simulink model "prova"  (R2018b)
settings: Solver=VariableStepAuto  StartTime=0.0  StopTime=inf  RelTol=1e-3
libraries: robotlib x3
settings Model: Creator=francesco  LastModifiedBy=francesco

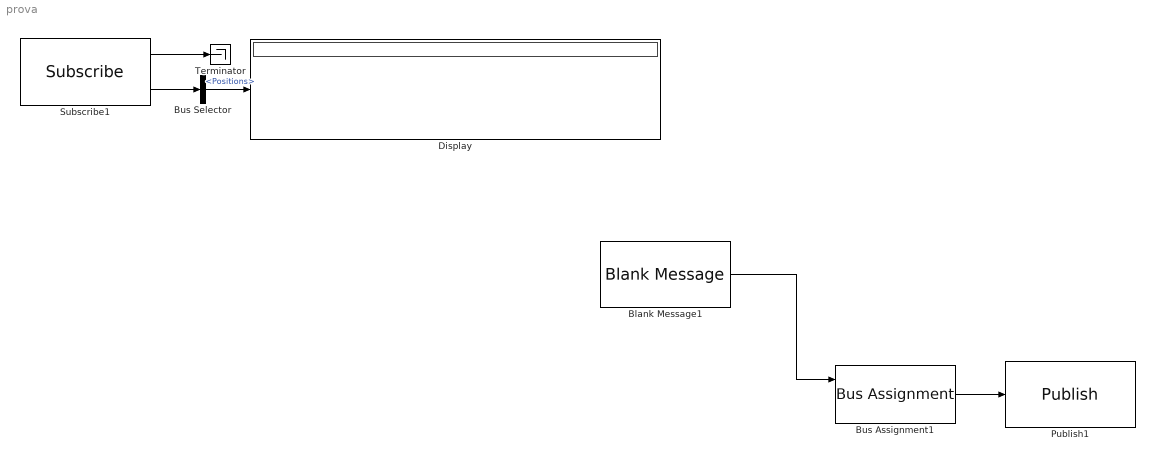
== system prova ==
  Blank Message1 : robotlib/Blank Message  messageClass=Message  entityType=std_msgs/Float64  messageType=std_msgs/Float64  SampleTime=-1
      settings: SourceProductBaseCode=RO
  Bus Assignment1 : BusAssignment  AssignedSignals=Data
  Bus Selector : BusSelector  OutputSignals=Actual.Positions
  Display : Display
  Publish1 : robotlib/Publish  topicSource=Select from ROS network  topic=/arm_controller/state  messageType=control_msgs/JointTrajectoryControllerState  messageQueueLength=1
      settings: SourceProductBaseCode=RO
  Subscribe1 : robotlib/Subscribe  topicSource=Select from ROS network  topic=/arm_controller/state  messageType=control_msgs/JointTrajectoryControllerState  sampleTime=-1  messageQueueLength=1
      settings: SourceProductBaseCode=RO
  Terminator : Terminator
  wires:
  Subscribe1/2 -> Bus Selector/1
  Subscribe1/1 -> Terminator/1
  Bus Assignment1/1 -> Publish1/1
  Blank Message1/1 -> Bus Assignment1/1
  Bus Selector/1 -> Display/1  "<Positions>"
